simulink model "W01_S2"  (R2024b)
settings: Solver=ode4  StartTime=0  StopTime=T_final  FixedStep=h  RelTol=1e-3
undefined symbols (not defined in the file or in its folder): beta_c, dn, mp, n0, rp, t_phase, V_c, x0
settings Model: Creator=admin  LastModifiedBy=admin
settings DataIOCC: ReturnWorkspaceOutputs=off

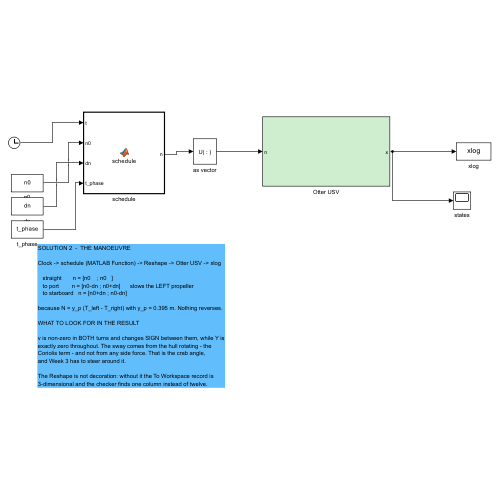
[thumbnail: Simulink's stored preview of the top-level diagram]
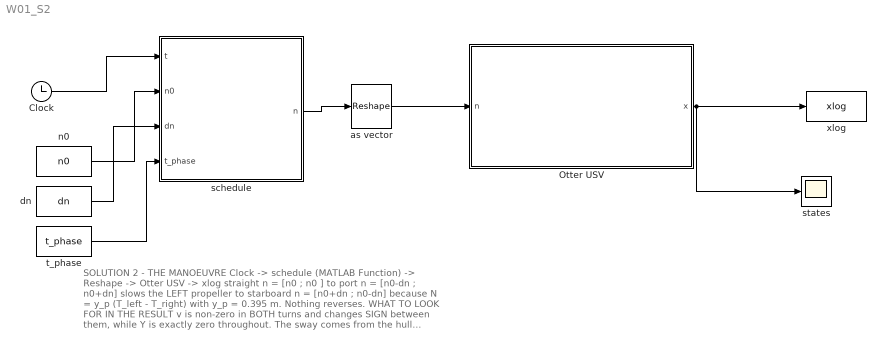
== system W01_S2 ==
  note: SOLUTION 2  -  THE MANOEUVRE
      |
      | Clock -> schedule (MATLAB Function) -> Reshape -> Otter USV -> xlog
      |
      |    straight       n = [n0    ; n0   ]
      |    to port        n = [n0-dn ; n0+dn]      slows the LEFT propeller
      |    to starboard   n = [n0+dn ; n0-dn]
      |
      | because N = y_p (T_left - T_right) with y_p = 0.395 m. Nothing reverses.
      |
      | WHAT TO LOOK FOR IN THE RESULT
      |
      | v is non-zero in BOTH turns and changes SIGN between them, while Y is
      | exactly zero throughout. The sway comes from the hull rotating - the
      | Coriolis term - and not from any side force. That is the crab angle,
      | and Week 3 has to steer around it.
      |
      | The Reshape is not decoration: without it the To Workspace record is
      | 3-dimensional and the checker finds one column instead of twelve.
  Clock : Clock
  Otter USV : Subsystem
  as vector : Reshape
  dn : Constant  Value=dn
  n0 : Constant  Value=n0
  schedule : MATLAB Function  TreatAsAtomicUnit=on
  states : Scope
  t_phase : Constant  Value=t_phase
  xlog : ToWorkspace  VariableName=xlog  SaveFormat=Structure With Time  SampleTime=-1
  wires:
  Clock/1 -> schedule/1(t)
  n0/1 -> schedule/2(n0)
  dn/1 -> schedule/3(dn)
  t_phase/1 -> schedule/4(t_phase)
  schedule/1(n) -> as vector/1
  as vector/1 -> Otter USV/1(n)
  Otter USV/1(x) -> xlog/1, states/1

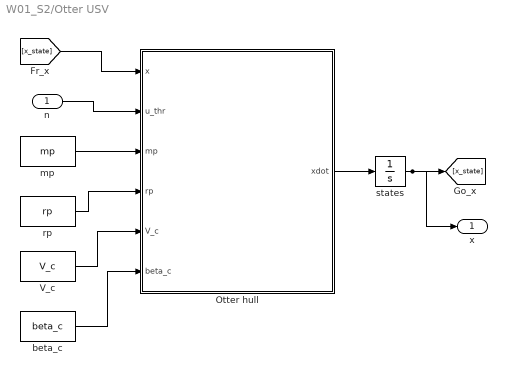
== system W01_S2/Otter USV ==
  n : Inport
  Otter hull : MATLAB Function  TreatAsAtomicUnit=on
  V_c : Constant  Value=V_c
  beta_c : Constant  Value=beta_c
  mp : Constant  Value=mp
  rp : Constant  Value=rp
  states : Integrator  InitialCondition=x0
  x : Outport
  wires:
  beta_c/1 -> Otter hull/6(beta_c)
  [x_state] -> Otter hull/1(x)
  V_c/1 -> Otter hull/5(V_c)
  n/1 -> Otter hull/2(u_thr)
  Otter hull/1(xdot) -> states/1
  mp/1 -> Otter hull/3(mp)
  rp/1 -> Otter hull/4(rp)
  states/1 -> x/1, [x_state]

== matlab function W01_S2/Otter USV/Otter hull ==
  data: x input; xdot output double size=[12 1]; u_thr input; mp input; rp input; V_c input; beta_c input
function xdot = otter_hull(x, u_thr, mp, rp, V_c, beta_c)
% Fossen's otter.m, called unchanged from Tools/MSS/VESSELS.
%
%   x       12 states, fed back from the integrator
%   u_thr   propeller shaft speeds [rad/s]
%
% otter.m is not written for code generation, so the call is extrinsic and
% xdot has to be pre-sized for Simulink to know the output width.
coder.extrinsic('otter');

xdot = zeros(12,1);
xdot = otter(x, u_thr, mp, rp, V_c, beta_c);
end

== matlab function W01_S2/schedule ==
  data: t input; n output double size=[2 1]; n0 input; dn input; t_phase input
function n = schedule(t, n0, dn, t_phase)
%#codegen
%SCHEDULE  Propeller command as a function of time.
%
%    straight -> port -> straight -> starboard -> straight
%
%  A turn is a DIFFERENCE between the two shaft speeds, because the yaw
%  moment is N = y_p (T_left - T_right). More thrust on the left turns the
%  bow to starboard, so a PORT turn slows the LEFT propeller.

nL = n0;  nR = n0;
if t >= t_phase(1) && t < t_phase(2)
    nL = n0 - dn;   nR = n0 + dn;      % port      (bow swings to -psi)
elseif t >= t_phase(3) && t < t_phase(4)
    nL = n0 + dn;   nR = n0 - dn;      % starboard (bow swings to +psi)
end
n = [nL; nR];
